simulink model "prob1"  (R2020a)
settings: Solver=VariableStepAuto  StartTime=0.0  StopTime=100  MaxStep=0.01  RelTol=1e-3
values from neighbouring files (symbols this model uses):
  A = 2.0    [data.sldd]    (also in parameter.m = 2)
  b = 50.0    [data.sldd]    (also in parameter.m = 50)
  k1 = 50.0    [data.sldd]    (also in parameter.m = 50)
  k12 = 500.0    [data.sldd]    (also in parameter.m = 500)
  M1 = 100.0    [data.sldd]    (also in parameter.m = 100)
  M2 = 5.0    [data.sldd]    (also in parameter.m = 5)
  w = 10.0    [data.sldd]    (also in parameter.m = 10)
settings Model: DataDictionary=data.sldd  Creator=Lenovo  LastModifiedBy=vijay

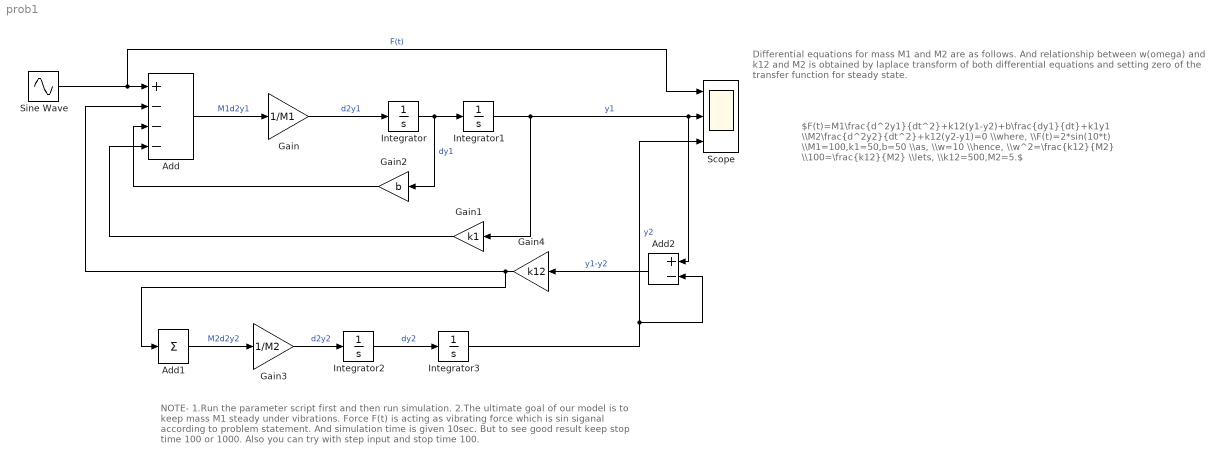
== system prob1 ==
  note: NOTE-
      | 1.Run the parameter script first and then run simulation.
      | 2.The ultimate goal of our model is to keep mass M1 steady under vibrations.
      | Force F(t) is acting as vibrating force which is sin siganal according to problem statement.
      | And simulation time is given 10sec. But to see good result keep stop time 100 or 1000.
      | Also you can try with step input and stop time 100.
  note: Differential equations for mass M1 and M2 are as follows.
      | And relationship between w(omega) and k12 and M2 is obtained by
      | laplace transform of both differential equations and setting zero
      | of the transfer function for steady state.
  note: $F(t)=M1\frac{d^2y1}{dt^2}+k12(y1-y2)+b\frac{dy1}{dt}+k1y1 \\M2\frac{d^2y2}{dt^2}+k12(y2-y1)=0 \\where, \\F(t)=2*sin(10*t) \\M1=100,k1=50,b=50 \\as, \\w=10 \\hence, \\w^2=\frac{k12}{M2} \\100=\frac{k12}{M2} \\lets, \\k12=500,M2=5.$
  Add : Sum  Inputs=+---
  Add1 : Sum  Inputs=+
  Add2 : Sum  Inputs=+-
  Gain : Gain  Gain=1/M1
  Gain1 : Gain  Gain=k1
  Gain2 : Gain  Gain=b
  Gain3 : Gain  Gain=1/M2
  Gain4 : Gain  Gain=k12
  Integrator{,1..3} (4 alike) : Integrator
  Scope : Scope  NumInputPorts=3
  Sine Wave : Sin  Amplitude=A  Frequency=w  SampleTime=0
  wires:
  Integrator/1 -> Gain2/1, Integrator1/1  "dy1"
  Gain/1 -> Integrator/1  "d2y1"
  Add/1 -> Gain/1  "M1d2y1"
  Integrator1/1 -> Add2/1, Scope/2, Gain1/1  "y1"
  Gain2/1 -> Add/3
  Gain1/1 -> Add/4
  Gain3/1 -> Integrator2/1  "d2y2"
  Integrator2/1 -> Integrator3/1  "dy2"
  Add1/1 -> Gain3/1  "M2d2y2"
  Integrator3/1 -> Add2/2, Scope/3  "y2"
  Add2/1 -> Gain4/1  "y1-y2"
  Gain4/1 -> Add1/1, Add/2
  Sine Wave/1 -> Scope/1, Add/1  "F(t)"
